simulink model "Andrew_squeezer_mechanism"  (R2015b)
settings: Solver=VariableStepAuto  StartTime=0.0  StopTime=.05  FixedStep=.05/100  RelTol=1e-3
InitFcn:
  | theta1=-0.06171; %(rad)
  | theta2=-0.3407950554; %(rad)
  | theta3=0.4880324482; %(rad)
  | theta4=-1.115516507; %(rad)
  | theta5=-1.350606450; %(rad)
  | theta6=1.350606450; %(rad)
  | theta7=-1.071524312; %(rad)
  | k_spring=4530; %(N/m)
  | l0=0.07785; %(m)
  | T=0.033; % (N.m)
  | beta0=-0.062; %(rad)
libraries: mblibv1 x36
settings Model: Creator=N56JN  LastModifiedBy=Asus
settings SimMechanicsCC: VisOnUpdateDiagram=on  VisDuringSimulation=on  LastVizWinPosition=[440.2 172.2 607.2 509.6]  CamPosition=[-0.036964;0.00375035;11.0557;]  CamTarget=[-0.036964;0.00375035;0;]  CamUpVector=[0;1;0;]  CamHeight=0.0754066  VisBackgroundColor=[0.9;0.9;0.95;]  DefaultBodyColor=[1;0;0;]  OVRRIDBodyVisualizationType=CONVHULL

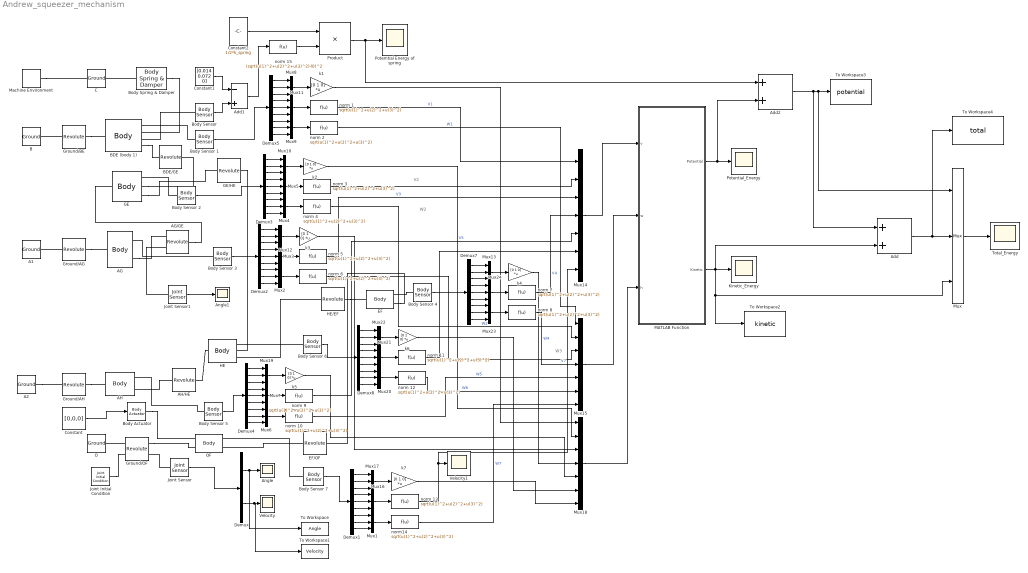
== system Andrew_squeezer_mechanism ==
  note: W3
  note: W2
  note: V2
  A1 : mblibv1/Bodies/Ground  UpdateFromCAD=off  LeftPortType=env  RightPortType=workingframe  PhysicalDomain=Mechanical  DialogClass=GroundBlock  CoordPosition=[-0.06934 -0.00227 0]  CoordPositionUnits=m  StateVectorMgrId=-1  MachineId=[0 0]  ShowEnvPort=off  ParameterChecksum=[0 0 0 0]  TopologyChecksum=[0 0 0 0]
  A2 : mblibv1/Bodies/Ground  UpdateFromCAD=off  LeftPortType=env  RightPortType=workingframe  PhysicalDomain=Mechanical  DialogClass=GroundBlock  CoordPosition=[-0.06934 -0.00227 0]  CoordPositionUnits=m  StateVectorMgrId=-1  MachineId=[0 0]  ShowEnvPort=off  ParameterChecksum=[0 0 0 0]  TopologyChecksum=[0 0 0 0]
  AG : mblibv1/Bodies/Body  LConnTagsString=CS1  RConnTagsString=CG|CS2  UpdateFromCAD=off  DialogClass=MechanicalBodyBlock  Mass=0.0705  MassUnits=kg  InertiaUnits=kg*m^2  Inertia=[0 0 0;0 0 0;0 0 1.169e-5]  Shape=Cylinder  ShapeDims=[1 1]  ShapeUnits=m  ShapeUse=false  Density=1  DensityUnits=kg/m^3  DensityUse=false  GraphicsMode=MACHINE_DEFAULT  BodyColorSelMode=MACHINE_DEFAULT  BodyColor=[1 0 0]  AttachedToCS=CG  CG=Right$CG$[0.02308 0.00916 0]$CS1$CS1$m$[0 0 0]$Euler X-Y-Z$rad$CS1$true$none  WorkingFrames=Left$CS1$[0 0 0]$Adjoining$Adjoining$m$[0 0 theta3]$Euler X-Y-Z$rad$Adjoining$true$none#Right$CS2$[0.04 0 0]$CS1$CS1$m$[0 0 0]$Euler X-Y-Z$rad$CS1$true$none  CGPos=[0.02308 0.00916 0]  CGRot=[0 0 0]  CS0Pos=[]  CS0Rot=[]  CS1Pos=[0 0 0]  CS1Rot=[0 0 theta3]  CS2Pos=[0.04 0 0]  CS2Rot=[0 0 0]  CS3Pos=[]  CS3Rot=[]  CS4Pos=[]  CS4Rot=[]  CS5Pos=[]  CS5Rot=[]  CS6Pos=[]  CS6Rot=[]  CS7Pos=[]  CS7Rot=[]  CS8Pos=[]  CS8Rot=[]  CS9Pos=[]  CS9Rot=[]  CS10Pos=[]  CS10Rot=[]  CS11Pos=[]  CS11Rot=[]  CS12Pos=[]  CS12Rot=[]  CS13Pos=[]  CS13Rot=[]  CS14Pos=[]  CS14Rot=[]  CS15Pos=[]  CS15Rot=[]  CS16Pos=[]  CS16Rot=[]  CS17Pos=[]  CS17Rot=[]  CS18Pos=[]  CS18Rot=[]  CS19Pos=[]  CS19Rot=[]  CS20Pos=[]  CS20Rot=[]
  AG/GE : mblibv1/Joints/Revolute  LConnTagsString=__newl0|SA1  RConnTagsString=__newr0  UpdateFromCAD=off  NumSAPorts=1  CutJoint=off  MarkAsCut=off  Primitives=prismatic  PrimitiveProps=R1$Base$[0 0 1]$revolute  DialogClass=JointBlock  R1Axis=[0 0 1]
  AH : mblibv1/Bodies/Body  LConnTagsString=CS1  RConnTagsString=CG|CS2  UpdateFromCAD=off  DialogClass=MechanicalBodyBlock  Mass=0.05498  MassUnits=kg  InertiaUnits=kg*m^2  Inertia=[0 0 0;0 0 0;0 0 1.912e-5]  Shape=Cylinder  ShapeDims=[1 1]  ShapeUnits=m  ShapeUse=false  Density=1  DensityUnits=kg/m^3  DensityUse=false  GraphicsMode=MACHINE_DEFAULT  BodyColorSelMode=MACHINE_DEFAULT  BodyColor=[1 0 0]  AttachedToCS=CG  CG=Right$CG$[0.01228 -0.00449 0]$CS1$CS1$m$[0 0 0]$Euler X-Y-Z$rad$CS1$true$none  WorkingFrames=Left$CS1$[0 0 0]$Adjoining$Adjoining$m$[0 0 theta2]$Euler X-Y-Z$rad$Adjoining$true$none#Right$CS2$[0.04 0 0]$CS1$CS1$m$[0 0 0]$Euler X-Y-Z$rad$CS1$true$none  CGPos=[0.01228 -0.00449 0]  CGRot=[0 0 0]  CS0Pos=[]  CS0Rot=[]  CS1Pos=[0 0 0]  CS1Rot=[0 0 theta2]  CS2Pos=[0.04 0 0]  CS2Rot=[0 0 0]  CS3Pos=[]  CS3Rot=[]  CS4Pos=[]  CS4Rot=[]  CS5Pos=[]  CS5Rot=[]  CS6Pos=[]  CS6Rot=[]  CS7Pos=[]  CS7Rot=[]  CS8Pos=[]  CS8Rot=[]  CS9Pos=[]  CS9Rot=[]  CS10Pos=[]  CS10Rot=[]  CS11Pos=[]  CS11Rot=[]  CS12Pos=[]  CS12Rot=[]  CS13Pos=[]  CS13Rot=[]  CS14Pos=[]  CS14Rot=[]  CS15Pos=[]  CS15Rot=[]  CS16Pos=[]  CS16Rot=[]  CS17Pos=[]  CS17Rot=[]  CS18Pos=[]  CS18Rot=[]  CS19Pos=[]  CS19Rot=[]  CS20Pos=[]  CS20Rot=[]
  AH/HE : mblibv1/Joints/Revolute  LConnTagsString=__newl0  RConnTagsString=__newr0  UpdateFromCAD=off  NumSAPorts=0  CutJoint=off  MarkAsCut=off  Primitives=prismatic  PrimitiveProps=R1$Base$[0 0 1]$revolute  DialogClass=JointBlock  R1Axis=[0 0 1]
  Add : Sum
  Add1 : Sum  Inputs=-+
  Add2 : Sum
  Angle : Scope
  Angle1 : Scope
  B : mblibv1/Bodies/Ground  UpdateFromCAD=off  LeftPortType=env  RightPortType=workingframe  PhysicalDomain=Mechanical  DialogClass=GroundBlock  CoordPosition=[-0.03635 0.03273 0]  CoordPositionUnits=m  StateVectorMgrId=-1  MachineId=[0 0]  ShowEnvPort=off  ParameterChecksum=[0 0 0 0]  TopologyChecksum=[0 0 0 0]
  BDE (body 1) : mblibv1/Bodies/Body  LConnTagsString=CS1  RConnTagsString=CG|CS3|CS2|CS4  UpdateFromCAD=off  DialogClass=MechanicalBodyBlock  Mass=0.02372  MassUnits=kg  InertiaUnits=kg*m^2  Inertia=[0 0 0;0 0 0;0 0 5.255e-6]  Shape=Cylinder  ShapeDims=[1 1]  ShapeUnits=m  ShapeUse=false  Density=1  DensityUnits=kg/m^3  DensityUse=false  GraphicsMode=MACHINE_DEFAULT  BodyColorSelMode=MACHINE_DEFAULT  BodyColor=[1 0 0]  AttachedToCS=CG  CG=Right$CG$[0.01874 0.01043 0]$CS1$CS1$m$[0 0 0]$Euler X-Y-Z$rad$CS1$true$none  WorkingFrames=Left$CS1$[0 0 0]$Adjoining$Adjoining$m$[0 0 theta4]$Euler X-Y-Z$rad$Adjoining$true$none#Right$CS3$[0.018 0.02 0]$CS1$CS1$m$[0 0 0]$Euler X-Y-Z$rad$CS1$true$none#Right$CS2$[0.018 0.02 0]$CS1$CS1$m$[0 0 0]$Euler X-Y-Z$rad$CS1$true$none#Right$CS4$[0.035 0 0]$CS1$CS1$m$[0 0 0]$Euler X-Y-Z$rad$CS1$true$none  CGPos=[0.01874 0.01043 0]  CGRot=[0 0 0]  CS0Pos=[]  CS0Rot=[]  CS1Pos=[0 0 0]  CS1Rot=[0 0 theta4]  CS2Pos=[0.018 0.02 0]  CS2Rot=[0 0 0]  CS3Pos=[0.018 0.02 0]  CS3Rot=[0 0 0]  CS4Pos=[0.035 0 0]  CS4Rot=[0 0 0]  CS5Pos=[]  CS5Rot=[]  CS6Pos=[]  CS6Rot=[]  CS7Pos=[]  CS7Rot=[]  CS8Pos=[]  CS8Rot=[]  CS9Pos=[]  CS9Rot=[]  CS10Pos=[]  CS10Rot=[]  CS11Pos=[]  CS11Rot=[]  CS12Pos=[]  CS12Rot=[]  CS13Pos=[]  CS13Rot=[]  CS14Pos=[]  CS14Rot=[]  CS15Pos=[]  CS15Rot=[]  CS16Pos=[]  CS16Rot=[]  CS17Pos=[]  CS17Rot=[]  CS18Pos=[]  CS18Rot=[]  CS19Pos=[]  CS19Rot=[]  CS20Pos=[]  CS20Rot=[]
  BDE/GE : mblibv1/Joints/Revolute  LConnTagsString=__newl0  RConnTagsString=__newr0  UpdateFromCAD=off  NumSAPorts=0  CutJoint=off  MarkAsCut=off  Primitives=prismatic  PrimitiveProps=R1$Base$[0 0 1]$revolute  DialogClass=JointBlock  R1Axis=[0 0 1]
  Body Actuator : mblibv1/Sensors &  Actuators/Body Actuator  UpdateFromCAD=off  PhysicalDomain=Mechanical  PortType=blob  ActuationStyle=Force  AngleUnits=deg  ArcVelocityUnits=deg/s  ArcAccelerationUnits=deg/s^2  CoordPositionUnits=m  VelocityUnits=m/s  AccelerationUnits=m/s^2  ForceUnits=N  TorqueUnits=N*m  ActiveIO=on  Width=3  DialogClass=MechanicalActuatorBlock  ReferenceFrame=Absolute (World)  Angle=off  CoordPosition=on  Force=off  Torque=on
  Body Sensor : mblibv1/Sensors &  Actuators/Body Sensor  UpdateFromCAD=off  PhysicalDomain=Mechanical  PortType=blob  Muxed=on  Pose=off  Angle=on  AngleUnits=deg  ArcVelocity=off  ArcVelocityUnits=deg/s  ArcAcceleration=off  ArcAccelerationUnits=deg/s^2  CoordPosition=on  CoordPositionUnits=m  Velocity=off  VelocityUnits=m/s  Acceleration=off  AccelerationUnits=m/s^2  Quaternion=on  QuaternionDT=off  QuaternionDDT=off  QuaternionUnits=off  OutputVector=[1]  ActiveIO=on  Width=3  DialogClass=MechanicalSensorBlock  ReferenceFrame=Absolute (World)
  Body Sensor {1..7} (7 alike) : mblibv1/Sensors &  Actuators/Body Sensor  UpdateFromCAD=off  PhysicalDomain=Mechanical  PortType=blob  Muxed=on  Pose=off  Angle=on  AngleUnits=deg  ArcVelocity=on  ArcVelocityUnits=rad/s  ArcAcceleration=off  ArcAccelerationUnits=deg/s^2  CoordPosition=on  CoordPositionUnits=m  Velocity=on  VelocityUnits=m/s  Acceleration=off  AccelerationUnits=m/s^2  Quaternion=on  QuaternionDT=off  QuaternionDDT=off  QuaternionUnits=off  OutputVector=[1]  ActiveIO=on  Width=9  DialogClass=MechanicalSensorBlock  ReferenceFrame=Absolute (World)
  Body Spring & Damper : mblibv1/Force  Elements/Body Spring & Damper  UpdateFromCAD=off  DialogClass=BodySpringDamper  Spring_k=k_spring  Damper_b=0  Offset_x0=l0  PositionUnits=m  VelocityUnits=m/s  ForceUnits=N
  C : mblibv1/Bodies/Ground  UpdateFromCAD=off  LeftPortType=env  RightPortType=workingframe  PhysicalDomain=Mechanical  DialogClass=GroundBlock  CoordPosition=[0.014 0.072 0]  CoordPositionUnits=m  StateVectorMgrId=0  MachineId=[1 0]  ShowEnvPort=on  ParameterChecksum=[2136964471, 472245319, 4220703987, 2520689520]  TopologyChecksum=[2000453322, 851108504, 435686989, 13641301]
  Constant : Constant  Value=[0,0,0]
  Constant1 : Constant  Value=[0.014 0.072 0]
  Constant2 : Constant  Value=1/2*k_spring
  Demux : Demux  Outputs=2
  Demux{1..5,7..8} (7 alike) : Demux  Outputs=9
  EF : mblibv1/Bodies/Body  LConnTagsString=CS1  RConnTagsString=CG|CS2  UpdateFromCAD=off  DialogClass=MechanicalBodyBlock  Mass=0.00365  MassUnits=kg  InertiaUnits=kg*m^2  Inertia=[0 0 0;0 0 0;0 0 4.41e-7]  Shape=Cylinder  ShapeDims=[1 1]  ShapeUnits=m  ShapeUse=false  Density=1  DensityUnits=kg/m^3  DensityUse=false  GraphicsMode=MACHINE_DEFAULT  BodyColorSelMode=MACHINE_DEFAULT  BodyColor=[1 0 0]  AttachedToCS=CG  CG=Right$CG$[0.0165 0 0]$CS1$CS1$m$[0 0 0]$Euler X-Y-Z$rad$CS1$true$none  WorkingFrames=Left$CS1$[0 0 0]$Adjoining$Adjoining$m$[0 0 theta7]$Euler X-Y-Z$rad$Adjoining$true$none#Right$CS2$[0.028 0 0]$CS1$CS1$m$[0 0 0]$Euler X-Y-Z$rad$CS1$true$none  CGPos=[0.0165 0 0]  CGRot=[0 0 0]  CS0Pos=[]  CS0Rot=[]  CS1Pos=[0 0 0]  CS1Rot=[0 0 theta7]  CS2Pos=[0.028 0 0]  CS2Rot=[0 0 0]  CS3Pos=[]  CS3Rot=[]  CS4Pos=[]  CS4Rot=[]  CS5Pos=[]  CS5Rot=[]  CS6Pos=[]  CS6Rot=[]  CS7Pos=[]  CS7Rot=[]  CS8Pos=[]  CS8Rot=[]  CS9Pos=[]  CS9Rot=[]  CS10Pos=[]  CS10Rot=[]  CS11Pos=[]  CS11Rot=[]  CS12Pos=[]  CS12Rot=[]  CS13Pos=[]  CS13Rot=[]  CS14Pos=[]  CS14Rot=[]  CS15Pos=[]  CS15Rot=[]  CS16Pos=[]  CS16Rot=[]  CS17Pos=[]  CS17Rot=[]  CS18Pos=[]  CS18Rot=[]  CS19Pos=[]  CS19Rot=[]  CS20Pos=[]  CS20Rot=[]
  EF/OF : mblibv1/Joints/Revolute  LConnTagsString=__newl0  RConnTagsString=__newr0  UpdateFromCAD=off  NumSAPorts=0  CutJoint=off  MarkAsCut=off  Primitives=prismatic  PrimitiveProps=R1$World$[0 0 1]$revolute  DialogClass=JointBlock  R1Axis=[0 0 1]
  GE : mblibv1/Bodies/Body  LConnTagsString=CS1  RConnTagsString=CG|CS2|CS3  UpdateFromCAD=off  DialogClass=MechanicalBodyBlock  Mass=0.00706  MassUnits=kg  InertiaUnits=kg*m^2  Inertia=[0 0 0;0 0 0;0 0 5.667e-7]  Shape=Cylinder  ShapeDims=[1 1]  ShapeUnits=m  ShapeUse=false  Density=1  DensityUnits=kg/m^3  DensityUse=false  GraphicsMode=MACHINE_DEFAULT  BodyColorSelMode=MACHINE_DEFAULT  BodyColor=[1 0 0]  AttachedToCS=CG  CG=Right$CG$[0.0058 0 0]$CS1$CS1$m$[0 0 0]$Euler X-Y-Z$rad$CS1$true$none  WorkingFrames=Left$CS1$[0 0 0]$Adjoining$Adjoining$m$[0 0 theta5]$Euler X-Y-Z$rad$Adjoining$true$none#Right$CS2$[0.02 0 0]$CS1$CS1$m$[0 0 0]$Euler X-Y-Z$rad$CS1$true$none#Right$CS3$[0.02 0 0]$CS1$CS1$m$[0 0 0]$Euler X-Y-Z$rad$CS1$true$none  CGPos=[0.0058 0 0]  CGRot=[0 0 0]  CS0Pos=[]  CS0Rot=[]  CS1Pos=[0 0 0]  CS1Rot=[0 0 theta5]  CS2Pos=[0.02 0 0]  CS2Rot=[0 0 0]  CS3Pos=[0.02 0 0]  CS3Rot=[0 0 0]  CS4Pos=[]  CS4Rot=[]  CS5Pos=[]  CS5Rot=[]  CS6Pos=[]  CS6Rot=[]  CS7Pos=[]  CS7Rot=[]  CS8Pos=[]  CS8Rot=[]  CS9Pos=[]  CS9Rot=[]  CS10Pos=[]  CS10Rot=[]  CS11Pos=[]  CS11Rot=[]  CS12Pos=[]  CS12Rot=[]  CS13Pos=[]  CS13Rot=[]  CS14Pos=[]  CS14Rot=[]  CS15Pos=[]  CS15Rot=[]  CS16Pos=[]  CS16Rot=[]  CS17Pos=[]  CS17Rot=[]  CS18Pos=[]  CS18Rot=[]  CS19Pos=[]  CS19Rot=[]  CS20Pos=[]  CS20Rot=[]
  GE/HE : mblibv1/Joints/Revolute  LConnTagsString=__newl0  RConnTagsString=__newr0  UpdateFromCAD=off  NumSAPorts=0  CutJoint=off  MarkAsCut=off  Primitives=prismatic  PrimitiveProps=R1$Base$[0 0 1]$revolute  DialogClass=JointBlock  R1Axis=[0 0 1]
  Ground/AG : mblibv1/Joints/Revolute  LConnTagsString=__newl0  RConnTagsString=__newr0  UpdateFromCAD=off  NumSAPorts=0  CutJoint=off  MarkAsCut=off  Primitives=prismatic  PrimitiveProps=R1$Base$[0 0 1]$revolute  DialogClass=JointBlock  R1Axis=[0 0 1]
  Ground/AH : mblibv1/Joints/Revolute  LConnTagsString=__newl0  RConnTagsString=__newr0  UpdateFromCAD=off  NumSAPorts=0  CutJoint=off  MarkAsCut=off  Primitives=prismatic  PrimitiveProps=R1$Base$[0 0 1]$revolute  DialogClass=JointBlock  R1Axis=[0 0 1]
  Ground/BE : mblibv1/Joints/Revolute  LConnTagsString=__newl0  RConnTagsString=__newr0  UpdateFromCAD=off  NumSAPorts=0  CutJoint=off  MarkAsCut=off  Primitives=prismatic  PrimitiveProps=R1$Base$[0 0 1]$revolute  DialogClass=JointBlock  R1Axis=[0 0 1]
  Ground/OF : mblibv1/Joints/Revolute  LConnTagsString=__newl0|SA1  RConnTagsString=__newr0|SA1  UpdateFromCAD=off  NumSAPorts=2  CutJoint=off  MarkAsCut=off  Primitives=prismatic  PrimitiveProps=R1$Base$[0 0 1]$revolute  DialogClass=JointBlock  R1Axis=[0 0 1]
  HE : mblibv1/Bodies/Body  LConnTagsString=CS1  RConnTagsString=CG|CS2|CS3  UpdateFromCAD=off  DialogClass=MechanicalBodyBlock  Mass=0.00706  MassUnits=kg  InertiaUnits=kg*m^2  Inertia=[0 0 0;0 0 0;0 0 5.667e-7]  Shape=Cylinder  ShapeDims=[1 1]  ShapeUnits=m  ShapeUse=false  Density=1  DensityUnits=kg/m^3  DensityUse=false  GraphicsMode=MACHINE_DEFAULT  BodyColorSelMode=MACHINE_DEFAULT  BodyColor=[1 0 0]  AttachedToCS=CG  CG=Right$CG$[0.0058 0 0]$CS1$CS1$m$[0 0 0]$Euler X-Y-Z$rad$CS1$true$none  WorkingFrames=Left$CS1$[0 0 0]$Adjoining$Adjoining$m$[0 0 theta6]$Euler X-Y-Z$rad$Adjoining$true$none#Right$CS2$[0.02 0 0]$CS1$CS1$m$[0 0 0]$Euler X-Y-Z$rad$CS1$true$none#Right$CS3$[0.02 0 0]$CS1$CS1$m$[0 0 0]$Euler X-Y-Z$rad$CS1$true$none  CGPos=[0.0058 0 0]  CGRot=[0 0 0]  CS0Pos=[]  CS0Rot=[]  CS1Pos=[0 0 0]  CS1Rot=[0 0 theta6]  CS2Pos=[0.02 0 0]  CS2Rot=[0 0 0]  CS3Pos=[0.02 0 0]  CS3Rot=[0 0 0]  CS4Pos=[]  CS4Rot=[]  CS5Pos=[]  CS5Rot=[]  CS6Pos=[]  CS6Rot=[]  CS7Pos=[]  CS7Rot=[]  CS8Pos=[]  CS8Rot=[]  CS9Pos=[]  CS9Rot=[]  CS10Pos=[]  CS10Rot=[]  CS11Pos=[]  CS11Rot=[]  CS12Pos=[]  CS12Rot=[]  CS13Pos=[]  CS13Rot=[]  CS14Pos=[]  CS14Rot=[]  CS15Pos=[]  CS15Rot=[]  CS16Pos=[]  CS16Rot=[]  CS17Pos=[]  CS17Rot=[]  CS18Pos=[]  CS18Rot=[]  CS19Pos=[]  CS19Rot=[]  CS20Pos=[]  CS20Rot=[]
  HE/EF : mblibv1/Joints/Revolute  LConnTagsString=__newl0  RConnTagsString=__newr0  UpdateFromCAD=off  NumSAPorts=0  CutJoint=off  MarkAsCut=off  Primitives=prismatic  PrimitiveProps=R1$Base$[0 0 1]$revolute  DialogClass=JointBlock  R1Axis=[0 0 1]
  Joint Initial Condition : mblibv1/Sensors &  Actuators/Joint Initial Condition  UpdateFromCAD=off  LeftPortType=blob  RightPortType=blob  PhysicalDomain=mechanical  DialogClass=InitialConditionBlock  InitialConditions=P1$false$0$m$deg$0$m/s$deg/s#P2$false$0$m$deg$0$m/s$deg/s#P3$false$0$m$deg$0$m/s$deg/s#R1$true$.06171$m$rad$0$m/s$rad/s#R2$false$0$m$deg$0$m/s$deg/s#R3$false$0$m$deg$0$m/s$deg/s#S$false$0$m$deg$0$m/s$deg/s  P1PIC=0  P1VIC=0  P2PIC=0  P2VIC=0  P3PIC=0  P3VIC=0  R1PIC=.06171  R1VIC=0  R2PIC=0  R2VIC=0  R3PIC=0  R3VIC=0  SPIC=0  SVIC=0
  Joint Sensor : mblibv1/Sensors &  Actuators/Joint Sensor  UpdateFromCAD=off  PhysicalDomain=Mechanical  PortType=blob  Muxed=on  Pose=off  Angle=on  AngleUnits=rad  ArcVelocity=on  ArcVelocityUnits=rad/s  ArcAcceleration=off  ArcAccelerationUnits=deg/s^2  CoordPosition=on  CoordPositionUnits=m  Velocity=off  VelocityUnits=m/s  Acceleration=off  AccelerationUnits=m/s^2  Quaternion=on  QuaternionDT=off  QuaternionDDT=off  QuaternionUnits=off  OutputVector=[1]  ActiveIO=on  Width=2  DialogClass=MechanicalSensorBlock  Primitive=R1  Force=off  ForceUnits=N  Torque=off  TorqueUnits=N*m  ReferenceFrame=Absolute (World)  ReactionSensedSide=Follower  ReactionReferenceFrame=Absolute (World)  ReactionForce=off  ReactionForceUnits=N  ReactionMoment=off  ReactionMomentUnits=N*m
  Joint Sensor1 : mblibv1/Sensors &  Actuators/Joint Sensor  UpdateFromCAD=off  PhysicalDomain=Mechanical  PortType=blob  Muxed=on  Pose=off  Angle=on  AngleUnits=rad  ArcVelocity=off  ArcVelocityUnits=rad/s  ArcAcceleration=off  ArcAccelerationUnits=deg/s^2  CoordPosition=on  CoordPositionUnits=m  Velocity=off  VelocityUnits=m/s  Acceleration=off  AccelerationUnits=m/s^2  Quaternion=on  QuaternionDT=off  QuaternionDDT=off  QuaternionUnits=off  OutputVector=[1]  ActiveIO=on  Width=1  DialogClass=MechanicalSensorBlock  Primitive=R1  Force=off  ForceUnits=N  Torque=off  TorqueUnits=N*m  ReferenceFrame=Absolute (World)  ReactionSensedSide=Follower  ReactionReferenceFrame=Absolute (World)  ReactionForce=off  ReactionForceUnits=N  ReactionMoment=off  ReactionMomentUnits=N*m
  Kinetic_Energy : Scope
  MATLAB Function : MATLAB Function  TreatAsAtomicUnit=on
  Machine Environment : mblibv1/Bodies/Machine Environment  PortType=env  PhysicalDomain=Mechanical  DialogTemplateClass=MECH.MachineEnvironment  SyncWhenCopied=off  Gravity=[0 -9.81 0]  GravityUnits=m/s^2  GravityAsSignal=off  Dimensionality=2D Only  AnalysisType=Forward dynamics  LinearAssemblyTolerance=1e-3  LinearAssemblyToleranceUnits=m  AngularAssemblyTolerance=1e-3  AngularAssemblyToleranceUnits=rad  ConstraintSolverType=Stabilizing  ConstraintRelTolerance=1e-4  ConstraintAbsTolerance=1e-4  UseRobustSingularityHandling=off  RedundancyAnalysisToleranceType=Automatically select tolerance  RedundancyAnalysisTolerance=1e-14  StatePerturbationType=Fixed  PerturbationSize=1e-5  VisualizeMachine=on  BodyVisualizationType=Use model default body geometries  BodyColorSelMode=Use model default  DefaultBodyColor=[1 0 0]
  Mux{,1..13,16..17,19..24} (22 alike) : Mux  Inputs=3
  Mux14 : Mux  Inputs=7
  Mux15 : Mux  Inputs=7
  Mux18 : Mux  Inputs=7
  O : mblibv1/Bodies/Ground  UpdateFromCAD=off  LeftPortType=env  RightPortType=workingframe  PhysicalDomain=Mechanical  DialogClass=GroundBlock  CoordPosition=[0 0 0]  CoordPositionUnits=m  StateVectorMgrId=-1  MachineId=[0 0]  ShowEnvPort=off  ParameterChecksum=[0 0 0 0]  TopologyChecksum=[0 0 0 0]
  OF : mblibv1/Bodies/Body  LConnTagsString=CS4|CS1  RConnTagsString=CG|CS2  UpdateFromCAD=off  DialogClass=MechanicalBodyBlock  Mass=0.04325  MassUnits=kg  InertiaUnits=kg*m^2  Inertia=[0 0 0;0 0 0;0 0 2.194e-6]  Shape=Cylinder  ShapeDims=[1 1]  ShapeUnits=m  ShapeUse=false  Density=1  DensityUnits=kg/m^3  DensityUse=false  GraphicsMode=MACHINE_DEFAULT  BodyColorSelMode=MACHINE_DEFAULT  BodyColor=[1 0 0]  AttachedToCS=CG  CG=Right$CG$[0.00092 0 0]$CS1$CS1$m$[0 0 0]$Euler X-Y-Z$rad$CS1$true$none  WorkingFrames=Left$CS4$[0.00092 0 0]$CS1$CS1$m$[0 0 0]$Euler X-Y-Z$rad$CS1$true$none#Left$CS1$[0 0 0]$Adjoining$Adjoining$m$[0 0 theta1]$Euler X-Y-Z$rad$Adjoining$true$none#Right$CS2$[0.007 0 0]$CS1$CS1$m$[0 0 0]$Euler X-Y-Z$rad$CS1$true$none  CGPos=[0.00092 0 0]  CGRot=[0 0 0]  CS0Pos=[]  CS0Rot=[]  CS1Pos=[0 0 0]  CS1Rot=[0 0 theta1]  CS2Pos=[0.007 0 0]  CS2Rot=[0 0 0]  CS3Pos=[]  CS3Rot=[]  CS4Pos=[0.00092 0 0]  CS4Rot=[0 0 0]  CS5Pos=[]  CS5Rot=[]  CS6Pos=[]  CS6Rot=[]  CS7Pos=[]  CS7Rot=[]  CS8Pos=[]  CS8Rot=[]  CS9Pos=[]  CS9Rot=[]  CS10Pos=[]  CS10Rot=[]  CS11Pos=[]  CS11Rot=[]  CS12Pos=[]  CS12Rot=[]  CS13Pos=[]  CS13Rot=[]  CS14Pos=[]  CS14Rot=[]  CS15Pos=[]  CS15Rot=[]  CS16Pos=[]  CS16Rot=[]  CS17Pos=[]  CS17Rot=[]  CS18Pos=[]  CS18Rot=[]  CS19Pos=[]  CS19Rot=[]  CS20Pos=[]  CS20Rot=[]
  Potemtial Energy of spring : Scope
  Potential_Energy : Scope
  Product : Product
  To Workspace : ToWorkspace  VariableName=Angle  SaveFormat=Timeseries  SampleTime=-1
  To Workspace1 : ToWorkspace  VariableName=Velocity  SaveFormat=Timeseries  SampleTime=-1
  To Workspace2 : ToWorkspace  VariableName=kinetic  SaveFormat=Timeseries  SampleTime=-1
  To Workspace3 : ToWorkspace  VariableName=potential  SaveFormat=Timeseries  SampleTime=-1
  To Workspace4 : ToWorkspace  VariableName=total  SaveFormat=Timeseries  SampleTime=-1
  Total_Energy : Scope
  Velocity : Scope
  Velocity1 : Scope
  k{1..7} (7 alike) : Gain  Gain=[0 1 0]  Multiplication=Matrix(K*u) (u vector)
  norm {1..13} (13 alike) : Fcn  Expr=sqrt(u(1)^2+u(2)^2+u(3)^2)
  norm 15 : Fcn  Expr=(sqrt(u(1)^2+u(2)^2+u(3)^2)-l0)^2
  norm14 : Fcn  Expr=sqrt(u(1)^2+u(2)^2+u(3)^2)
  wires:
  Joint Sensor/1 -> Demux/1
  Demux/1 -> To Workspace/1, Angle/1
  Demux/2 -> To Workspace1/1, Velocity/1
  Body Sensor 7/1 -> Demux1/1
  Mux1/1 -> norm14/1
  Body Sensor 6/1 -> Demux8/1
  Body Sensor 4/1 -> Demux7/1
  Body Sensor 5/1 -> Demux4/1
  Body Sensor 1/1 -> Demux5/1
  Body Sensor 2/1 -> Demux3/1
  norm 1/1 -> Mux14/1  "V1"
  norm 5/1 -> Mux14/3  "V3"
  norm 7/1 -> Mux14/4  "V4"
  norm 9/1 -> Mux14/5  "V5"
  norm 11/1 -> Mux14/6
  Mux14/1 -> MATLAB Function/1(v)
  Mux15/1 -> MATLAB Function/2(w)
  norm14/1 -> Mux15/7  "W7"
  norm 12/1 -> Mux15/6  "W6"
  norm 10/1 -> Mux15/5  "W5"
  norm 8/1 -> Mux15/4  "W4"
  norm 6/1 -> Mux15/3
  norm 4/1 -> Mux15/2  "W2"
  norm 2/1 -> Mux15/1  "W1"
  norm 3/1 -> Mux14/2
  norm 13/1 -> Mux14/7, Velocity1/1  "V7"
  Demux1/1 -> Mux17/1
  Demux1/2 -> Mux17/2
  Demux1/3 -> Mux17/3
  Demux1/4 -> Mux16/1
  Demux1/5 -> Mux16/2
  Demux1/6 -> Mux16/3
  Demux1/7 -> Mux1/1
  Demux1/8 -> Mux1/2
  Demux1/9 -> Mux1/3
  Mux16/1 -> norm 13/1
  Mux17/1 -> k7/1
  k7/1 -> Mux18/7
  Mux6/1 -> norm 10/1
  Demux4/1 -> Mux19/1
  Demux4/2 -> Mux19/2
  Demux4/3 -> Mux19/3
  Demux4/4 -> Mux7/1
  Demux4/5 -> Mux7/2
  Demux4/6 -> Mux7/3
  Demux4/7 -> Mux6/1
  Demux4/8 -> Mux6/2
  Demux4/9 -> Mux6/3
  Mux7/1 -> norm 9/1
  Mux19/1 -> k5/1
  k5/1 -> Mux18/5
  Mux20/1 -> norm 12/1
  Demux8/1 -> Mux22/1
  Demux8/2 -> Mux22/2
  Demux8/3 -> Mux22/3
  Demux8/4 -> Mux21/1
  Demux8/5 -> Mux21/2
  Demux8/6 -> Mux21/3
  Demux8/7 -> Mux20/1
  Demux8/8 -> Mux20/2
  Demux8/9 -> Mux20/3
  Mux21/1 -> norm 11/1
  Mux22/1 -> k6/1
  k6/1 -> Mux18/6
  Mux2/1 -> norm 6/1
  Demux2/1 -> Mux12/1
  Demux2/2 -> Mux12/2
  Demux2/3 -> Mux12/3
  Demux2/4 -> Mux3/1
  Demux2/5 -> Mux3/2
  Demux2/6 -> Mux3/3
  Demux2/7 -> Mux2/1
  Demux2/8 -> Mux2/2
  Mux3/1 -> norm 5/1
  Mux12/1 -> k3/1
  Body Sensor 3/1 -> Demux2/1
  k3/1 -> Mux18/3
  Mux23/1 -> norm 8/1
  Demux7/1 -> Mux13/1
  Demux7/2 -> Mux13/2
  Demux7/3 -> Mux13/3
  Demux7/4 -> Mux24/1
  Demux7/5 -> Mux24/2
  Demux7/6 -> Mux24/3
  Demux7/7 -> Mux23/1
  Demux7/8 -> Mux23/2
  Mux24/1 -> norm 7/1
  Mux13/1 -> k4/1
  k4/1 -> Mux18/4
  Mux4/1 -> norm 4/1
  Demux3/1 -> Mux10/1
  Demux3/2 -> Mux10/2
  Demux3/3 -> Mux10/3
  Demux3/4 -> Mux5/1
  Demux3/5 -> Mux5/2
  Demux3/6 -> Mux5/3
  Demux3/7 -> Mux4/1
  Demux3/8 -> Mux4/2
  Demux3/9 -> Mux4/3
  Mux5/1 -> norm 3/1
  k2/1 -> Mux18/2
  Mux9/1 -> norm 2/1
  Demux5/1 -> Mux8/1
  Demux5/2 -> Mux8/2
  Demux5/3 -> Mux8/3
  Demux5/4 -> Mux11/1
  Demux5/5 -> Mux11/2
  Demux5/6 -> Mux11/3
  Demux5/7 -> Mux9/1
  Demux5/8 -> Mux9/2
  Demux5/9 -> Mux9/3
  Mux11/1 -> norm 1/1
  Mux8/1 -> k1/1
  k1/1 -> Mux18/1
  Mux18/1 -> MATLAB Function/3(h)
  Demux2/9 -> Mux2/3
  Constant/1 -> Body Actuator/1
  Joint Sensor1/1 -> Angle1/1
  Mux10/1 -> k2/1
  Body Sensor/1 -> Add1/2
  Constant1/1 -> Add1/1
  Add1/1 -> norm 15/1
  Constant2/1 -> Product/1
  norm 15/1 -> Product/2
  Demux7/9 -> Mux23/3
  Add/1 -> To Workspace4/1, Mux/2
  Mux/1 -> Total_Energy/1
  Product/1 -> Add2/1, Potemtial Energy of spring/1
  MATLAB Function/1(Potential) -> Potential_Energy/1, Add2/2
  MATLAB Function/2(Kinetic) -> Add/2, Mux/3, To Workspace2/1, Kinetic_Energy/1
  Add2/1 -> Add/1, Mux/1, To Workspace3/1
  connections:
  Ground/AG/RConn1 -- AG/LConn1
  GE/HE/RConn1 -- HE/RConn2
  Ground/OF/RConn1 -- OF/LConn2
  Ground/BE/RConn1 -- BDE (body 1)/LConn1
  EF/RConn2 -- EF/OF/RConn1
  Body Spring & Damper/RConn1 -- BDE (body 1)/RConn2
  AH/HE/RConn1 -- HE/LConn1
  Ground/AG/LConn1 -- A1/RConn1
  AH/HE/LConn1 -- AH/RConn2
  AG/RConn2 -- AG/GE/LConn1
  HE/EF/LConn1 -- HE/RConn3
  Ground/AH/RConn1 -- AH/LConn1
  Ground/BE/LConn1 -- B/RConn1
  Joint Sensor/LConn1 -- Ground/OF/RConn2
  EF/OF/LConn1 -- OF/RConn2
  GE/RConn3 -- GE/HE/LConn1
  HE/EF/RConn1 -- EF/LConn1
  Joint Initial Condition/RConn1 -- Ground/OF/LConn2
  A2/RConn1 -- Ground/AH/LConn1
  Body Spring & Damper/LConn1 -- C/RConn1
  AG/GE/RConn1 -- GE/LConn1
  Joint Sensor1/LConn1 -- AG/GE/LConn2
  Ground/OF/LConn1 -- O/RConn1
  Machine Environment/RConn1 -- C/LConn1
  GE/RConn2 -- BDE/GE/RConn1
  BDE (body 1)/RConn4 -- BDE/GE/LConn1
  Body Sensor 5/LConn1 -- AH/RConn1
  Body Sensor 3/LConn1 -- AG/RConn1
  Body Sensor 1/LConn1 -- BDE (body 1)/RConn1
  Body Sensor 2/LConn1 -- GE/RConn1
  Body Sensor 4/LConn1 -- EF/RConn1
  Body Sensor 6/LConn1 -- HE/RConn1
  Body Sensor 7/LConn1 -- OF/RConn1
  Body Actuator/RConn1 -- OF/LConn1
  Body Sensor/LConn1 -- BDE (body 1)/RConn3

== matlab function Andrew_squeezer_mechanism/MATLAB Function ==
  data: Potential output; v input; Kinetic output; w input; h input
function [Potential,Kinetic] = fcn(v,w,h)
% cd('E:\paper');
m1=0.02373;
I1=5.255e-6;
m2=0.00706;
I2=5.667e-7;
m3=0.0705;
I3=1.169e-5;
m4=0.00365;
I4=4.41e-7;
m5=0.05498;
I5=1.912e-5;
m6=0.00706;
I6=5.667e-7;
m7=0.04325;
I7=2.194e-6;
g=9.81;

m=[m1,m2,m3,m4,m5,m6,m7];
I=[I1,I2,I3,I4,I5,I6,I7];

Kinetic=0;
Potential=0;
for i=1:7
    Kinetic=Kinetic+0.5*(m(i)*v(i)^2+I(i)*w(i)^2);
    Potential=Potential+m(i)*g*h(i);
end
